simulink model "sys2"  (R2017b)
settings: Solver=VariableStepAuto  StartTime=0.0  StopTime=10  RelTol=1e-3
values from neighbouring files (symbols this model uses):
  Cs2 = tf([5 50],[1])    [main.m]
  Fs2 = tf([10],[1 10])    [main.m]
  Gs_Ident = tf([-0.009224 6.08],[1 1.241 1.475])    [main.m]
libraries: simulink x1
settings Model: Creator=Matheus  LastModifiedBy=Matheus

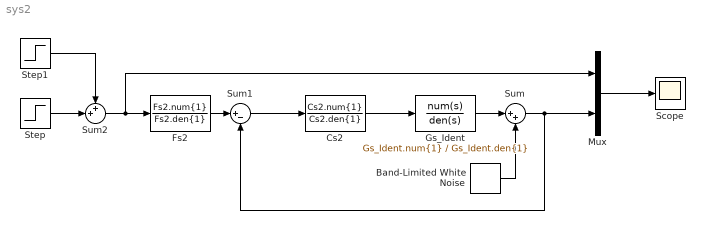
== system sys2 ==
  Band-Limited White Noise : simulink/Sources/Band-Limited White Noise  Cov=1e-7  Ts=1e-3  seed=[23341]
  Cs2 : TransferFcn  Numerator=Cs2.num{1}  Denominator=Cs2.den{1}
  "Fs2 " : TransferFcn  Numerator=Fs2.num{1}  Denominator=Fs2.den{1}
  Gs_Ident : TransferFcn  Numerator=Gs_Ident.num{1}  Denominator=Gs_Ident.den{1}
  Mux : Mux  Inputs=2
  Scope : Scope
  Step : Step  SampleTime=0
  Step1 : Step  SampleTime=5
  Sum : Sum  Inputs=|++
  Sum1 : Sum  Inputs=|+-
  Sum2 : Sum  Inputs=++|
  wires:
  Cs2/1 -> Gs_Ident/1
  Step/1 -> Sum2/2
  Sum/1 -> Sum1/2, Mux/2
  Mux/1 -> Scope/1
  Band-Limited White Noise/1 -> Sum/2
  "Fs2 "/1 -> Sum1/1
  Sum2/1 -> Mux/1, "Fs2 "/1
  Step1/1 -> Sum2/1
  Sum1/1 -> Cs2/1
  Gs_Ident/1 -> Sum/1
